simulink model "lin_modell_laufk_und_winkel"  (R2016b)
settings: Solver=FixedStepAuto  StartTime=0.0  StopTime=15  RelTol=1e-3
undefined symbols (not defined in the file or in its folder): param
libraries: simulink_extras x2
settings Model: Creator=Patrick  LastModifiedBy=Fritz

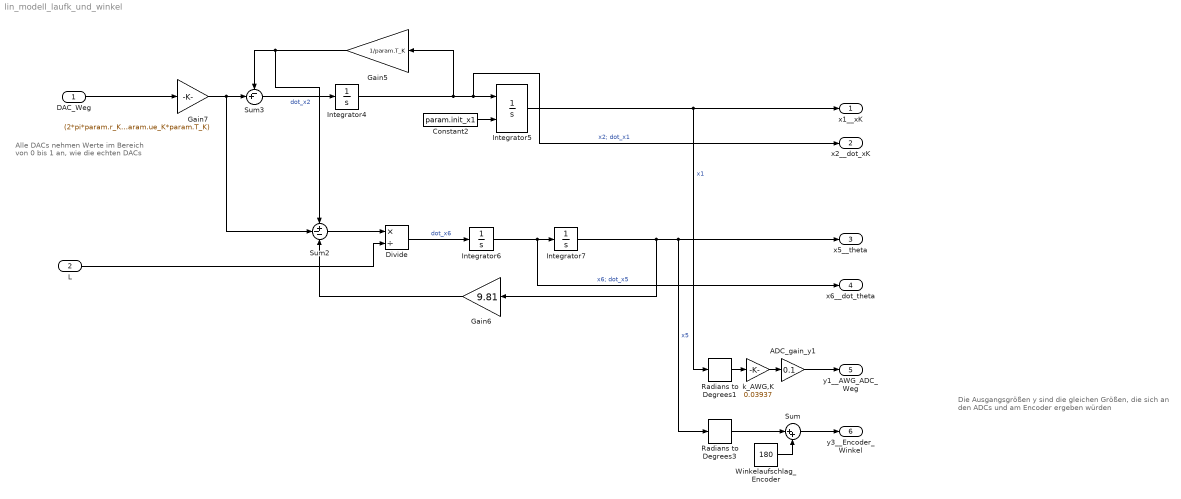
== system lin_modell_laufk_und_winkel ==
  note: Die Ausgangsgrößen y sind die gleichen Größen,
      | die sich an den ADCs und am Encoder ergeben würden
  note: Alle DACs nehmen Werte im Bereich
      | von 0 bis 1 an, wie die echten DACs
  DAC_Weg : Inport
  L : Inport  Port=2
  ADC_gain_y1 : Gain  Gain=0.1
  Constant2 : Constant  Value=param.init_x1
  Divide : Product  Inputs=*/
  Gain5 : Gain  Gain=1/param.T_K
  Gain6 : Gain  Gain=9.81
  Gain7 : Gain  Gain=(2*pi*param.r_K*param.K_K)/(param.ue_K*param.T_K)
  Integrator4 : Integrator
  Integrator5 : Integrator  InitialConditionSource=external
  Integrator6 : Integrator
  Integrator7 : Integrator
  Radians to Degrees1 : simulink_extras/Transformations/Radians to Degrees
  Radians to Degrees3 : simulink_extras/Transformations/Radians to Degrees
  Sum : Sum  Inputs=|++
  Sum2 : Sum  Inputs=+--
  Sum3 : Sum  Inputs=-+|
  Winkelaufschlag_Encoder : Constant  Value=180
  k_AWG,K : Gain  Gain=0.03937
  x1__xK : Outport  SignalName=x1__xK
  x2__dot_xK : Outport  Port=2  SignalName=x2__dot_xK
  x5__theta : Outport  Port=3  SignalName=x5__theta
  x6__dot_theta : Outport  Port=4  SignalName=x6__dot_theta
  y1__AWG_ADC_Weg : Outport  Port=5  SignalName=y1__AWG_ADC_Weg
  y3__Encoder_Winkel : Outport  Port=6  SignalName=y3__Encoder_Winkel
  wires:
  k_AWG,K/1 -> ADC_gain_y1/1
  Winkelaufschlag_Encoder/1 -> Sum/2
  Sum/1 -> y3__Encoder_Winkel/1
  ADC_gain_y1/1 -> y1__AWG_ADC_Weg/1
  DAC_Weg/1 -> Gain7/1
  Sum3/1 -> Integrator4/1  "dot_x2"
  Integrator4/1 -> x2__dot_xK/1, Integrator5/1, Gain5/1  "x2; dot_x1"
  Gain5/1 -> Sum2/1, Sum3/1
  Constant2/1 -> Integrator5/2
  Gain7/1 -> Sum2/2, Sum3/2
  Sum2/1 -> Divide/1
  Divide/1 -> Integrator6/1  "dot_x6"
  Integrator6/1 -> x6__dot_theta/1, Integrator7/1  "x6; dot_x5"
  Integrator7/1 -> x5__theta/1, Radians to Degrees3/1, Gain6/1  "x5"
  Gain6/1 -> Sum2/3
  Integrator5/1 -> Radians to Degrees1/1, x1__xK/1  "x1"
  L/1 -> Divide/2
  Radians to Degrees1/1 -> k_AWG,K/1
  Radians to Degrees3/1 -> Sum/1
